simulink model "BatteryFastCharging"  (R2026a)
settings: Solver=ode15s  StopTime=4000  MaxStep=10  RelTol=1e-4
InitFcn:
  | spm_path__ = 'BatteryFastCharging/BatteryPlant/SPM';
  | F__ = 96485;
  | L_a__ = str2double(get_param(spm_path__, 'ThicknessAnode'));
  | L_c__ = str2double(get_param(spm_path__, 'ThicknessCathode'));
  | A__ = str2double(get_param(spm_path__, 'ElectrodePlateArea'));
  | eps_a__ = str2double(get_param(spm_path__, 'ActiveMaterialVolumeFractionAnode'));
  | eps_c__ = str2double(get_param(spm_path__, 'ActiveMaterialVolumeFractionCathode'));
  | c_max_a__ = str2double(get_param(spm_path__, 'MaximumConcentrationAnode'));
  | c_max_c__ = str2double(get_param(spm_path__, 'MaximumConcentrationCathode'));
  | theta_max_a__ = str2double(get_param(spm_path__, 'MaximumStoichiometryAnode'));
  | theta_min_a__ = str2double(get_param(spm_path__, 'MinimumStoichiometryAnode'));
  | theta_max_c__ = str2double(get_param(spm_path__, 'MaximumStoichiometryCathode'));
  | theta_min_c__ = str2double(get_param(spm_path__, 'MinimumStoichiometryCathode'));
  | Q_nom = min(eps_a__*L_a__*A__*c_max_a__*(theta_max_a__ - theta_min_a__), ...
  |             eps_c__*L_c__*A__*c_max_c__*(theta_max_c__ - theta_min_c__)) * F__ / 3600;
  | clear spm_path__ F__ L_a__ L_c__ A__ eps_a__ eps_c__ c_max_a__ c_max_c__ theta_max_a__ theta_min_a__ theta_max_c__ theta_min_c__;
values from neighbouring files (symbols this model uses):
  active_controller = 1    [setupParams.m]
  c_s_anode_max = 24344    [setupParams.m]
  I_charge = Q_nom    (= 5)    [setupParams.m]
  Kp_cv = 10    [setupParams.m]
  ms_currents = [2*Q_nom, 1.5*Q_nom, 1*Q_nom]    [setupParams.m]
  ms_soc_thresholds = [0.5, 0.7, SOC_target]    [setupParams.m]
  SOC_init = 0.2    [setupParams.m]
  SOC_target = 0.9    [setupParams.m]
  T_ambient = 298.15    [setupParams.m]
  T_max = 323.15    [setupParams.m]
  V_max = 4.2    [setupParams.m]
libraries: fl_lib x6, nesl_utility x4, BatteryEstimators x1, batt_lib x1, BatteryCurrentManagement x1
settings Model: SimulationMode=accelerator  Creator=rvalenti  LastModifiedBy=rvalenti

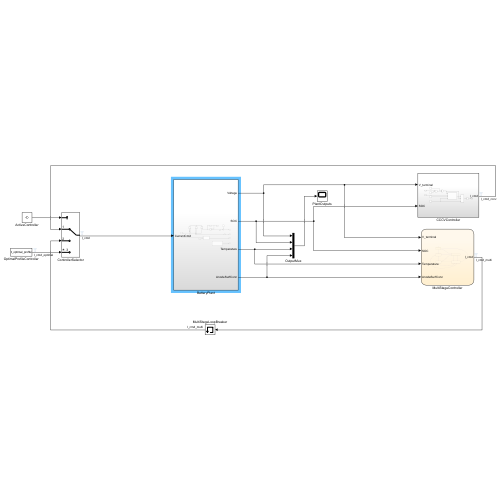
[thumbnail: Simulink's stored preview of the top-level diagram]
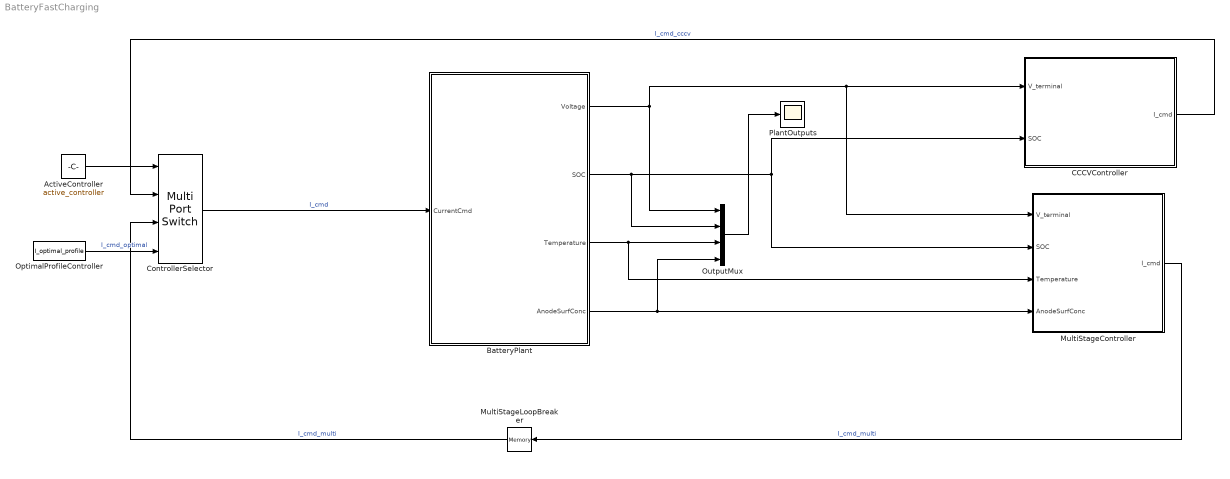
== system BatteryFastCharging ==
  ActiveController : Constant  Value=active_controller
  BatteryPlant : Subsystem
  CCCVController : Subsystem
  ControllerSelector : MultiPortSwitch  DataPortOrder=Specify indices
  MultiStageController : Stateflow chart  TreatAsAtomicUnit=on
  MultiStageLoopBreaker : Memory
  OptimalProfileController : FromWorkspace  VariableName=I_optimal_profile  SampleTime=0.1  OutputAfterFinalValue=Setting to zero
  OutputMux : Mux
  PlantOutputs : Scope
  wires:
  BatteryPlant/1(Voltage) -> MultiStageController/1(V_terminal), CCCVController/1(V_terminal), OutputMux/1
  BatteryPlant/2(SOC) -> CCCVController/2(SOC), MultiStageController/2(SOC), OutputMux/2
  BatteryPlant/3(Temperature) -> OutputMux/3, MultiStageController/3(Temperature)
  BatteryPlant/4(AnodeSurfConc) -> OutputMux/4, MultiStageController/4(AnodeSurfConc)
  OutputMux/1 -> PlantOutputs/1
  MultiStageController/1(I_cmd) -> MultiStageLoopBreaker/1  "I_cmd_multi"
  ActiveController/1 -> ControllerSelector/1
  CCCVController/1(I_cmd) -> ControllerSelector/2  "I_cmd_cccv"
  MultiStageLoopBreaker/1 -> ControllerSelector/3  "I_cmd_multi"
  OptimalProfileController/1 -> ControllerSelector/4  "I_cmd_optimal"
  ControllerSelector/1 -> BatteryPlant/1(CurrentCmd)  "I_cmd"

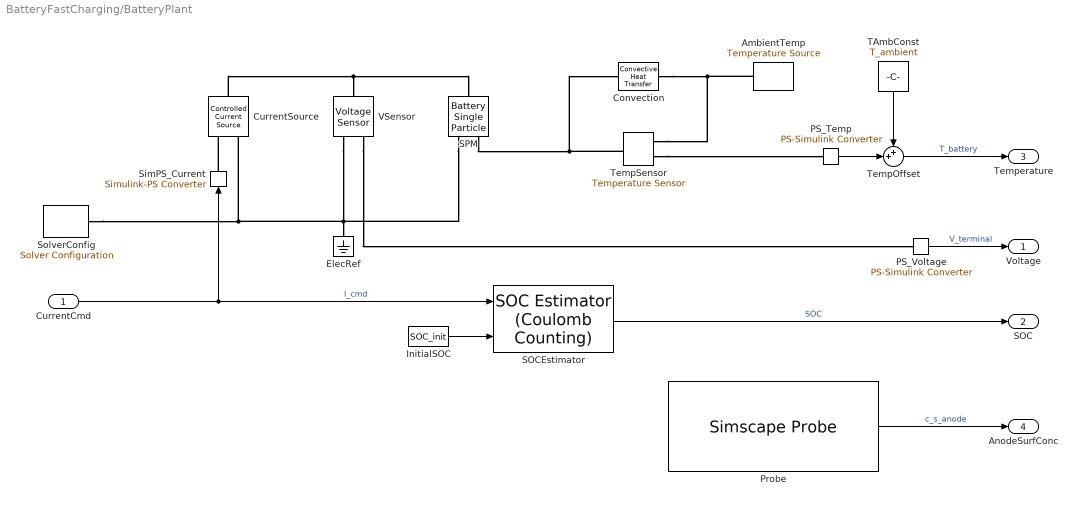
== system BatteryFastCharging/BatteryPlant ==
  CurrentCmd : Inport
  AmbientTemp : fl_lib/Thermal/Thermal Sources/Temperature Source  temperature=T_ambient K
  Convection : fl_lib/Thermal/Thermal Elements/Convective Heat Transfer  thermal_type=foundation.enum.constant_variable.constant  area=A_cell m^2  heat_tr_coeff=h_conv W/(K*m^2)  min_heat_tr_coeff=1e-3 W/(K*m^2)  T_specify=off  T_priority=None  T=0 K  T_nominal_specify=off  T_nominal_value=1  T_nominal_unit=K  Q_specify=off  Q_priority=None  Q=0 W  Q_nominal_specify=off  Q_nominal_value=1  Q_nominal_unit=W
  CurrentSource : fl_lib/Electrical/Electrical Sources/Controlled Current Source
  ElecRef : fl_lib/Electrical/Electrical Elements/Electrical Reference
  InitialSOC : Constant  Value=SOC_init
  PS_Temp : nesl_utility/PS-Simulink Converter  PhysicalDomain=network_engine_domain  SubClassName=ps_output  LeftPortType=input  RightPortType=output  PseudoPeriodic=off  Frequencies=[]  VectorFormat=inherit  Unit=K  AffineConversion=off
  PS_Voltage : nesl_utility/PS-Simulink Converter  PhysicalDomain=network_engine_domain  SubClassName=ps_output  LeftPortType=input  RightPortType=output  PseudoPeriodic=off  Frequencies=[]  VectorFormat=inherit  Unit=V  AffineConversion=off
  Probe : SimscapeProbe  BoundBlock=9  Variables="{\"anodeModel.surfaceConcentration\":{\"Probing\":\"ON\"}}"
  SOCEstimator : BatteryEstimators/SOC Estimator (Coulomb Counting)  CurrentInputPartition=on  AH=Q_nom  Ts=-1  DataType=Inherit: auto
  SPM : batt_lib/Cells/Electrochemical/Battery Single Particle  ExtrapolationMethod=simscape.enum.extrapolation.nearest  ThicknessAnode=3.4E-5 m  ElectrolyteLayerCountAnode=10  ThicknessSeparator=2.5E-5 m  ElectrolyteLayerCountSeparator=5  ThicknessCathode=8E-5 m  ElectrolyteLayerCountCathode=10  ElectrodePlateArea=0.39 m^2  ParticleRadiusAnode=5E-6 m  ShellCountAnode=10  ParticleRadiusCathode=5E-8 m  ShellCountCathode=10  ActiveMaterialVolumeFractionAnode=0.58  ActiveMaterialVolumeFractionCathode=0.374  StoichiometryBreakpointsSpecification=simscape.battery.enum.cells.electrochemical.StoichiometryBreakpointsSpecification.normalized  NormalizedStoichiometryBreakpoints=linspace(0.025, 0.975, 39)  OpenCircuitPotentialAnode=[.435; .325; .259; .221; .204; .194; .179; .166; .155; .145; .137; .131; .128; .127; .126; .125; .124; .123; .122; .121; .118; .117; .112; .109; .105; .1; .098; .095; .094; .093; .091; .09; .089; .088; .087; .086; .085; .084; .083] V  OpenCircuitPotentialCathode=[3.598; 3.53; 3.494; 3.474; 3.46; 3.455; 3.454; 3.453; 3.4528; 3.4526; 3.4524; 3.452; 3.4518; 3.4516; 3.4514; 3.4512; 3.451; 3.4508; 3.4506; 3.4503; 3.45; 3.4498; 3.4495; 3.4493; 3.449; 3.4488; 3.4486; 3.4484; 3.4482; 3.4479; 3.4477; 3.4475; 3.4473; 3.447; 3.4468; 3.4466; 3.4464; 3.4462; 3.4458] V  AbsoluteStoichiometryBreakpointsAnode=linspace(0.025, 0.975, 39)  OpenCircuitPotentialAbsoluteAnode=[.484; .335; .253; .209; .2; .181; .165; .151; .139; .131; .128; .125; .124; .124; .123; .122; .119; .117; .111; .108; .101; .098; .095; .093; .092; .088; .088; .088; .088; .087; .087; .087; .085; .082; .079; .071; .064; .049; .026] V  AbsoluteStoichiometryBreakpointsCathode=linspace(0.025, 0.975, 39)  OpenCircuitPotentialAbsoluteCathode=[3.81; 3.608; 3.512; 3.478; 3.459; 3.453; 3.45257; 3.45214; 3.45171; 3.45128; 3.45085; 3.45042; 3.44999; 3.44956; 3.44913; 3.4487; 3.44827; 3.44784; 3.44741; 3.44698; 3.44655; 3.44612; 3.44569; 3.44526; 3.44483; 3.4444; 3.44397; 3.44354; 3.44311; 3.44268; 3.44225; 3.44182; 3.44139; 3.44096; 3.44053; 3.44; 3.412; 3.304; 2.968] V  MaximumConcentrationAnode=30555 mol/m^3  MaximumStoichiometryAnode=0.811  MinimumStoichiometryAnode=0.0132  MaximumConcentrationCathode=22806 mol/m^3  MaximumStoichiometryCathode=0.74  MinimumStoichiometryCathode=0.035  ActiveMaterialDiffusionCoefficientAnode=6E-15 m^2/s  ActiveMaterialDiffusionCoefficientCathode=3.0E-19 m^2/s  ConductivityAnode=100 S/m  ConductivityCathode=0.5 S/m  CurrentCollectorResistance=0 Ohm  ElectrolyteVolumeFractionAnode=0.3874  ElectrolyteVolumeFractionSeparator=0.45  ElectrolyteVolumeFractionCathode=0.5725  ElectrolyteConductivity=0.85 S/m  BruggemanExponentAnode=1.5  BruggemanExponentSeparator=1.5  BruggemanExponentCathode=1.5  TransferenceNumber=0.363  ElectrolyteDiffusionCoefficient=3.5E-10 m^2/s  ChargeTransferRateAnode=8.8E-14 m^(5/2)/(mol^(1/2)*s)  ChargeTransferRateCathode=2.8E-13 m^(5/2)/(mol^(1/2)*s)  BatteryThermalMass=45 J/K  ArrheniusReferenceTemperature=298.15 K  ActiveMaterialDiffusionActivationEnergyAnode=39000 J/mol  ActiveMaterialDiffusionActivationEnergyCathode=35000 J/mol  ElectrolyteDiffusionActivationEnergy=26600 J/mol  ConductivityActivationEnergyAnode=3000 J/mol  ConductivityActivationEnergyCathode=3000 J/mol  ElectrolyteConductivityActivationEnergy=11000 J/mol  ChargeTransferActivationEnergyAnode=13000 J/mol  ChargeTransferActivationEnergyCathode=20000 J/mol  InnerSEIMethod=simscape.battery.enum.cells.electrochemical.InnerSEIMethod.none  MolarVolumeInnerSEI=5E-3 m^3/mol  DiffusionCoefficientInnerSEI=1E-20 m^2/s  StoichiometricCoefficientInnerSEI=2  DiffusionActivationEnergyInnerSEI=39000 J/mol  ConductivityInnerSEI=5.0E-6 S/m  ConductivityActivationEnergyInnerSEI=39000 J/mol  PlatingMethod=simscape.battery.enum.cells.electrochemical.PlatingMethod.none  ExchangeCurrentDensityPlating=3E-4 A/m^2  ActivationEnergyPlating=3000 J/mol  ReversibilityFactorPlating=0.5  batteryCurrent_specify=off  batteryCurrent_priority=None  batteryCurrent=0 A  batteryCurrent_nominal_specify=off  batteryCurrent_nominal_value=1  batteryCurrent_nominal_unit=A  batteryVoltage_specify=off  batteryVoltage_priority=None  batteryVoltage=0 V  batteryVoltage_nominal_specify=off  batteryVoltage_nominal_value=1  batteryVoltage_nominal_unit=V  averageElectrolyteConcentration_specify=on  averageElectrolyteConcentration_priority=High  averageElectrolyteConcentration=1500 mol/m^3  averageElectrolyteConcentration_nominal_specify=off  averageElectrolyteConcentration_nominal_value=1  averageElectrolyteConcentration_nominal_unit=mol/m^3  stateOfCharge_specify=on  stateOfCharge_priority=High  stateOfCharge=SOC_init  stateOfCharge_nominal_specify=off  stateOfCharge_nominal_value=1  stateOfCharge_nominal_unit=1  batteryTemperature_specify=on  batteryTemperature_priority=High  batteryTemperature=T_init K  batteryTemperature_nominal_specify=off  batteryTemperature_nominal_value=1  batteryTemperature_nominal_unit=K  thicknessSEI_specify=off  thicknessSEI_priority=High  thicknessSEI=1E-7 m  thicknessSEI_nominal_specify=off  thicknessSEI_nominal_value=1  thicknessSEI_nominal_unit=m  reversiblePlatedMaterial_specify=off  reversiblePlatedMaterial_priority=High  reversiblePlatedMaterial=0 mol  reversiblePlatedMaterial_nominal_specify=off  reversiblePlatedMaterial_nominal_value=1  reversiblePlatedMaterial_nominal_unit=mol  irreversiblePlatedMaterial_specify=off  irreversiblePlatedMaterial_priority=High  irreversiblePlatedMaterial=0 mol  irreversiblePlatedMaterial_nominal_specify=off  irreversiblePlatedMaterial_nominal_value=1  irreversiblePlatedMaterial_nominal_unit=mol  power_dissipated_specify=off  power_dissipated_priority=None  power_dissipated=0 W  power_dissipated_nominal_specify=off  power_dissipated_nominal_value=1  power_dissipated_nominal_unit=W  heatGenerationRate_specify=off  heatGenerationRate_priority=None  heatGenerationRate=0 W  heatGenerationRate_nominal_specify=off  heatGenerationRate_nominal_value=1  heatGenerationRate_nominal_unit=W
  SimPS_Current : nesl_utility/Simulink-PS Converter  PhysicalDomain=network_engine_domain  SubClassName=ps_input  LeftPortType=input  RightPortType=output  PseudoPeriodic=off  Frequencies=[]  NoiseDistribution=none  NoiseParameters=[]  Unit=1  AffineConversion=off  FilteringAndDerivatives=provide  SimscapeFilterOrder=1  InputFilterTimeConstant=0.001  UdotUserProvided=0
  SolverConfig : nesl_utility/Solver Configuration  PhysicalDomain=network_engine_domain  SubClassName=solver  LeftPortType=input  RightPortType=generic  Tones=[]  Harmonics=[]  SimulateNoise=off  Profile=off  UseLocalSampling=off  EnableSwitchedLinearOptims=on  FrequencyDomain=off  UseCCode=off  RelTol=0.001  AbsTol=0.001  MinStep=1e-09  ToWorkspace=off  RevertToSquareIcSolve=off  NumHomotopyIterations=100  PhasorMode=off  PhasorModeNumHarmonics=1  ConsistencySolver=NEWTON_XTOL_AFTER_FTOL  CanonicalOrdering=CANONICAL  OptimizeIntermediates=OPTIMIZED  IndexReductionMethod=DerivativeReplacement  DoDC=off  ResidualTolerance=1e-09  ConsistencyTolSource=GLOBAL  ConsistencyAbsTol=0.001  ConsistencyRelTol=0.001  ConsistencyTolFactor=0.001  UseLocalSolver=off  LocalSolverChoice=NE_BACKWARD_EULER_ADVANCER  ResolveIndetEquations=on  FunctionEvalNumThread=1  LocalSolverSampleTime=0.001  DoFixedCost=off  MaxNonlinIter=3  MaxModeIter=2  ComputeImpulses=off  ImpulseIterations=2  LinearAlgebra=auto  LinearAlgebraNumThread=0  EquationFormulation=NE_TIME_EF  DelaysMemoryBudget=1024  AutomaticFiltering=on  FilteringTimeConstant=0.001  PartitionStorageMethod=AS_NEEDED  PartitionMemoryBudget=1024  PartitionMethod=ROBUST  MultibodyUseLocalSolver=off  MultibodyLocalSolverChoice=ODE1  MultibodyLocalSolverSampleTime=0.001
  TAmbConst : Constant  Value=T_ambient
  TempOffset : Sum  Inputs=++|
  TempSensor : fl_lib/Thermal/Thermal Sensors/Temperature Sensor  temperature_measure=foundation.enum.MeasurementReference.difference
  VSensor : fl_lib/Electrical/Electrical Sensors/Voltage Sensor
  Voltage : Outport
  SOC : Outport  Port=2
  Temperature : Outport  Port=3
  AnodeSurfConc : Outport  Port=4
  wires:
  CurrentCmd/1 -> SOCEstimator/1, SimPS_Current/1  "I_cmd"
  PS_Voltage/1 -> Voltage/1  "V_terminal"
  TempOffset/1 -> Temperature/1  "T_battery"
  PS_Temp/1 -> TempOffset/2
  TAmbConst/1 -> TempOffset/1
  InitialSOC/1 -> SOCEstimator/2
  SOCEstimator/1 -> SOC/1  "SOC"
  Probe/1 -> AnodeSurfConc/1  "c_s_anode"
  connections:
  SimPS_Current/RConn1 -- CurrentSource/RConn1
  CurrentSource/LConn1 -- SPM/LConn1 -- VSensor/LConn1
  SPM/RConn1 -- ElecRef/LConn1 -- VSensor/RConn2 -- CurrentSource/RConn2 -- SolverConfig/RConn1
  VSensor/RConn1 -- PS_Voltage/LConn1
  SPM/RConn2 -- TempSensor/LConn1 -- Convection/LConn1
  TempSensor/RConn1 -- AmbientTemp/LConn1 -- Convection/RConn1
  TempSensor/RConn2 -- PS_Temp/LConn1

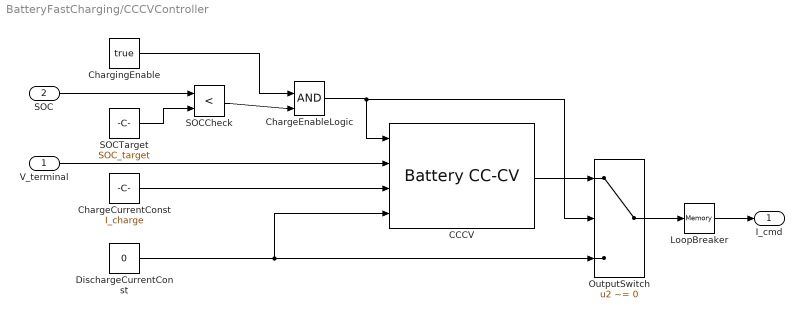
== system BatteryFastCharging/CCCVController ==
  V_terminal : Inport
  SOC : Inport  Port=2
  CCCV : BatteryCurrentManagement/Battery CC-CV  MinMaxFlag=off  MaxCellVoltage=V_max  Kp=100  Ki=10  Kaw=1  Kt=1  Ts=0.1
  ChargeCurrentConst : Constant  Value=I_charge
  ChargeEnableLogic : Logic  IconShape=distinctive  AllPortsSameDT=off  OutDataTypeStr=boolean
  ChargingEnable : Constant  Value=true  OutDataTypeStr=boolean
  DischargeCurrentConst : Constant  Value=0
  LoopBreaker : Memory  InitialCondition=I_charge
  OutputSwitch : Switch  Criteria=u2 ~= 0
  SOCCheck : RelationalOperator  Operator=<
  SOCTarget : Constant  Value=SOC_target
  I_cmd : Outport
  wires:
  SOC/1 -> SOCCheck/1
  SOCTarget/1 -> SOCCheck/2
  ChargingEnable/1 -> ChargeEnableLogic/1
  SOCCheck/1 -> ChargeEnableLogic/2
  ChargeEnableLogic/1 -> OutputSwitch/2, CCCV/1
  V_terminal/1 -> CCCV/2
  ChargeCurrentConst/1 -> CCCV/3
  DischargeCurrentConst/1 -> CCCV/4, OutputSwitch/3
  CCCV/1 -> OutputSwitch/1
  OutputSwitch/1 -> LoopBreaker/1
  LoopBreaker/1 -> I_cmd/1

== stateflow chart BatteryFastCharging/MultiStageController ==
  settings: updateMethod=DISCRETE  sampleTime=0.1
  state Stage1
    entry: I_cmd = ms_currents(1);
  state CV
    during: I_cmd = max(0, Kp_cv * (V_max - V_terminal));
  state Stage2
    entry: I_cmd = ms_currents(2);
  state Stage3
    entry: I_cmd = ms_currents(3);
  state Done
    entry: I_cmd = 0;
  (default) -> Stage1
  Stage1 -> Done [order 3] : [Temperature >= T_max || AnodeSurfConc >= c_s_anode_max]
  Stage1 -> CV [order 2] : [V_terminal >= V_max]
  Stage1 -> Stage2 [order 1] : [SOC >= ms_soc_thresholds(1)]
  Stage2 -> CV [order 2] : [V_terminal >= V_max]
  Stage2 -> Done [order 3] : [Temperature >= T_max || AnodeSurfConc >= c_s_anode_max]
  Stage3 -> CV [order 2] : [V_terminal >= V_max]
  CV -> Done [order 1] : [SOC >= ms_soc_thresholds(3)]
  CV -> Done [order 2] : [Temperature >= T_max || AnodeSurfConc >= c_s_anode_max]
  Stage2 -> Stage3 [order 1] : [SOC >= ms_soc_thresholds(2)]
  Stage3 -> Done [order 3] : [Temperature >= T_max || AnodeSurfConc >= c_s_anode_max]
  Stage3 -> Done [order 1] : [SOC >= ms_soc_thresholds(3)]
  data: V_terminal input; SOC input; Temperature input; AnodeSurfConc input; I_cmd output; ms_currents parameter; ms_soc_thresholds parameter; V_max parameter; Kp_cv parameter; T_max parameter; c_s_anode_max parameter
